simulink library "INT_ExtDem_CalcState"  (R2016b)
settings: Solver=VariableStepAuto  StartTime=0.0  StopTime=10.0  RelTol=1e-3
settings Model: Creator=xuxingpei  LastModifiedBy=xuxingpei

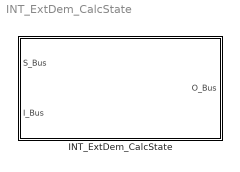
== system INT_ExtDem_CalcState ==
  INT_ExtDem_CalcState : Subsystem

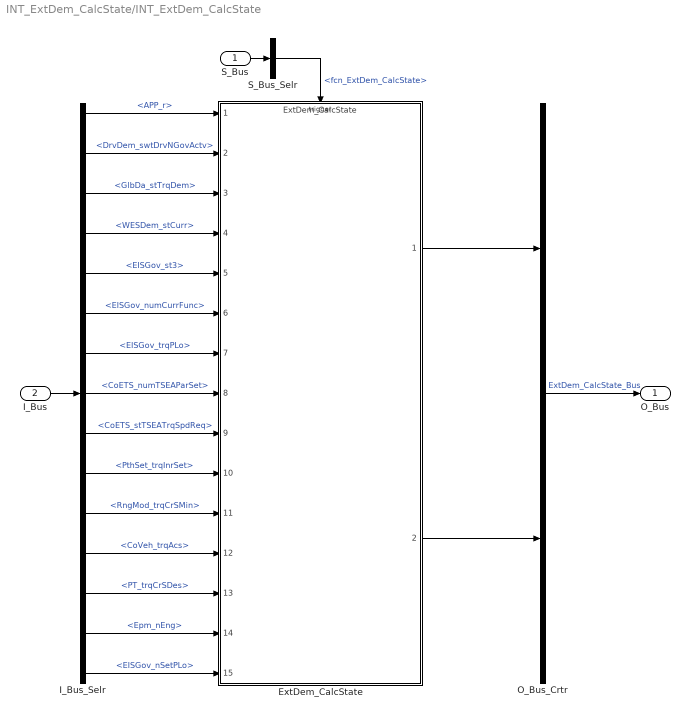
== system INT_ExtDem_CalcState/INT_ExtDem_CalcState ==
  S_Bus : Inport
  I_Bus : Inport  Port=2
  ExtDem_CalcState : ModelReference  ModelNameDialog=ExtDem_CalcState  SimulationMode=Normal  ModelReferenceVersion=1.15  TriggerPortName=function  TriggerPortTriggerType=function-call  TriggerPortStatesWhenEnabling=held
  I_Bus_Selr : BusSelector  OutputSignals=APP_r,DrvDem_swtDrvNGovActv,GlbDa_stTrqDem,WESDem_stCurr,EISGov_st3,EISGov_numCurrFunc,EISGov_trqPLo,CoETS_numTSEAParSet,CoETS_stTSEATrqSpdReq,PthSet_trqInrSet,RngMod_trqCrSMin,CoVeh_trqAcs,PT_trqCrSDes,Epm_nEng,EISGov_nSetPLo
  O_Bus_Crtr : BusCreator  Inputs=2
  S_Bus_Selr : BusSelector  OutputSignals=fcn_ExtDem_CalcState
  O_Bus : Outport
  wires:
  S_Bus_Selr/1 -> ExtDem_CalcState/Trigger  "<fcn_ExtDem_CalcState>"
  S_Bus/1 -> S_Bus_Selr/1
  I_Bus/1 -> I_Bus_Selr/1
  I_Bus_Selr/1 -> ExtDem_CalcState/1  "<APP_r>"
  I_Bus_Selr/2 -> ExtDem_CalcState/2  "<DrvDem_swtDrvNGovActv>"
  I_Bus_Selr/3 -> ExtDem_CalcState/3  "<GlbDa_stTrqDem>"
  I_Bus_Selr/4 -> ExtDem_CalcState/4  "<WESDem_stCurr>"
  I_Bus_Selr/5 -> ExtDem_CalcState/5  "<EISGov_st3>"
  I_Bus_Selr/6 -> ExtDem_CalcState/6  "<EISGov_numCurrFunc>"
  I_Bus_Selr/7 -> ExtDem_CalcState/7  "<EISGov_trqPLo>"
  I_Bus_Selr/8 -> ExtDem_CalcState/8  "<CoETS_numTSEAParSet>"
  I_Bus_Selr/9 -> ExtDem_CalcState/9  "<CoETS_stTSEATrqSpdReq>"
  I_Bus_Selr/10 -> ExtDem_CalcState/10  "<PthSet_trqInrSet>"
  I_Bus_Selr/11 -> ExtDem_CalcState/11  "<RngMod_trqCrSMin>"
  I_Bus_Selr/12 -> ExtDem_CalcState/12  "<CoVeh_trqAcs>"
  I_Bus_Selr/13 -> ExtDem_CalcState/13  "<PT_trqCrSDes>"
  I_Bus_Selr/14 -> ExtDem_CalcState/14  "<Epm_nEng>"
  I_Bus_Selr/15 -> ExtDem_CalcState/15  "<EISGov_nSetPLo>"
  O_Bus_Crtr/1 -> O_Bus/1  "ExtDem_CalcState_Bus"
  ExtDem_CalcState/1 -> O_Bus_Crtr/1
  ExtDem_CalcState/2 -> O_Bus_Crtr/2
